simulink model "population_control_model"  (R2014b)
settings: Solver=ode45  StartTime=0.0  StopTime=30  RelTol=1e-3
libraries: simulink x1
settings Model: Creator=Shane Reynolds  LastModifiedBy=Shane Reynolds

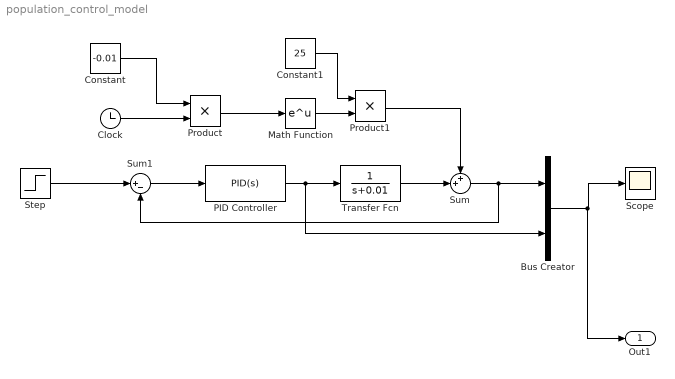
== system population_control_model ==
  Bus Creator : BusCreator  Inputs=2
  Clock : Clock
  Constant : Constant  Value=-0.01
  Constant1 : Constant  Value=25
  Math Function : Math  SaturateOnIntegerOverflow=on
  PID Controller : simulink/Continuous/PID Controller  Controller=PID  TimeDomain=Continuous-time  SampleTime=-1  IntegratorMethod=Forward Euler  FilterMethod=Forward Euler  Form=Parallel  P=1.2  I=0.001  D=0.1  N=0.378094165182863  InitialConditionSource=internal  InitialConditionForIntegrator=0  InitialConditionForFilter=0  ExternalReset=none  LimitOutput=on  UpperSaturationLimit=0.75  LowerSaturationLimit=0  LinearizeAsGain=on  AntiWindupMode=none  Kb=1  TrackingMode=off  Kt=1  PParamMin=[]  PParamMax=[]  IParamMin=[]  IParamMax=[]  DParamMin=[]  DParamMax=[]  NParamMin=[]  NParamMax=[]  KbParamMin=[]  KbParamMax=[]  KtParamMin=[]  KtParamMax=[]  POutMin=[]  POutMax=[]  IOutMin=[]  IOutMax=[]  DOutMin=[]  DOutMax=[]  NOutMin=[]  NOutMax=[]  KbOutMin=[]  KbOutMax=[]  KtOutMin=[]  KtOutMax=[]  IntegratorOutMin=[]  IntegratorOutMax=[]  FilterOutMin=[]  FilterOutMax=[]  SumOutMin=[]  SumOutMax=[]  SumI1OutMin=[]  SumI1OutMax=[]  SumI2OutMin=[]  SumI2OutMax=[]  SumI3OutMin=[]  SumI3OutMax=[]  SumDOutMin=[]  SumDOutMax=[]  SaturationOutMin=[]  SaturationOutMax=[]  IntegratorContinuousStateAttributes=''  IntegratorStateMustResolveToSignalObject=off  IntegratorRTWStateStorageClass=Auto  FilterContinuousStateAttributes=''  FilterStateMustResolveToSignalObject=off  FilterRTWStateStorageClass=Auto  DifferentiatorICPrevScaledInput=0  DifferentiatorOutMin=[]  DifferentiatorOutMax=[]  UseFilter=on
  Product : Product
  Product1 : Product
  Scope : Scope
      settings: ScrollMode=on
  Step : Step  Time=0  Before=25  After=20  SampleTime=0
  Sum : Sum  Inputs=++|
  Sum1 : Sum  Inputs=|+-
  Transfer Fcn : TransferFcn  Denominator=[1 0.01]
  Out1 : Outport
  wires:
  PID Controller/1 -> Bus Creator/2, Transfer Fcn/1
  Sum1/1 -> PID Controller/1
  Step/1 -> Sum1/1
  Clock/1 -> Product/2
  Product/1 -> Math Function/1
  Constant/1 -> Product/1
  Math Function/1 -> Product1/2
  Transfer Fcn/1 -> Sum/2
  Sum/1 -> Bus Creator/1, Sum1/2
  Product1/1 -> Sum/1
  Constant1/1 -> Product1/1
  Bus Creator/1 -> Out1/1, Scope/1
